simulink model "CEL_Lab1_Feedforward"  (R2024b)
settings: Solver=ode45  StartTime=0.0  StopTime=5
values from neighbouring files (symbols this model uses):
  PID = computePIDGains(8, 0.15, 0.1, plant.Ps, "PID")    [lab1_startup.m]
undefined symbols (not defined in the file or in its folder): drv, gbox, mld, mot, rads2rpm, sens
libraries: simulink_extras x3
settings Model: Creator=bmm1  LastModifiedBy=bmm1
settings RTWCC: GPUComputeCapability=3.5

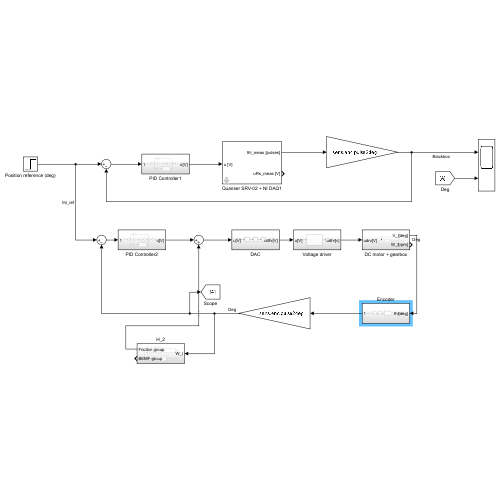
[thumbnail: Simulink's stored preview of the top-level diagram]
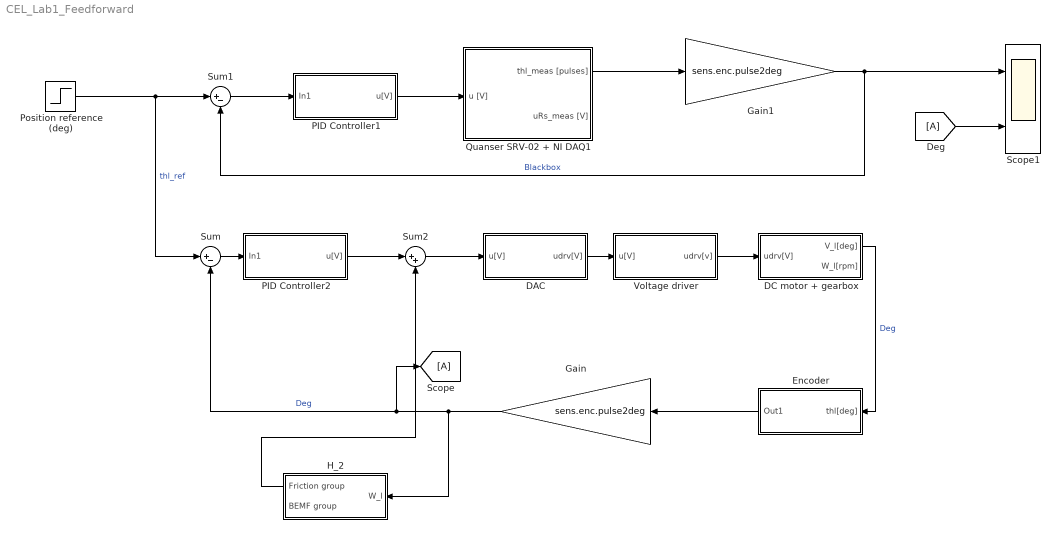
== system CEL_Lab1_Feedforward ==
  DAC : Subsystem
  DC motor + gearbox : Subsystem
  Deg : From
  Encoder : Subsystem
  Gain : Gain  Gain=sens.enc.pulse2deg
  Gain1 : Gain  Gain=sens.enc.pulse2deg
  H_2 : Subsystem
  PID Controller1 : Subsystem
  PID Controller2 : Subsystem
  Position reference (deg) : Step  Time=0.5  After=360  SampleTime=0
  Quanser SRV-02 + NI DAQ1 : Subsystem  mask(Quanser SRV-02 (with inertial load) + NI DAQ){Ts=0.001, fricType=Coulomb + viscous}
      mask prompts: Ts "NI DAQ Sample Time:"; fricType "Friction model"
      mask help: Quanser SRV-02 (with inertial load) + NI DAQ model.
      mask init:
      | %%  Sensors data
      | 
      | %   shunt resistor
      | sens.curr.Rs = 0.5;                         %   resistance [Ohm]   
      | sens.curr.uRs_std = 0.01;                   %   voltage noise standard dev [V]                           
      | sens.curr.uRs_var = sens.curr.uRs_std^2;	%   voltage noise variance [V^2]
      | 
      | %   Hewlett-Packard HEDS-5540#A06 optical encoder
      | sens.enc.ppr = 500*4;                       %   pulses per rotation
      | sens.enc.pulse2deg = 360/sens.enc.ppr;      %   [pulses] -> [deg]
      | sens.enc.pulse2rad = 2*pi/sens.enc.ppr;     %   [pulses] -> [rad]
      | sens.enc.deg2pulse = sens.enc.ppr/360;      %   [deg] -> [pulses]
      | sens.enc.rad2pulse = sens.enc.ppr/2/pi;     %   [rad] -> [pulses]
      | 
      | 
      | %%  Data acquisition board (daq) data
      | 
      | %   NI PCI-6221 DAC data
      | daq.dac.bits = 16;                                  %   resolution (bits)
      | daq.dac.fs   = 10;                                  %   full scale 
      | daq.dac.q    = 2*daq.dac.fs/(2^daq.dac.bits-1);     %	quantization
      | 
      | %   NI PCI-6221 ADC data
      | daq.adc.bits = 16;                                  %   resolution (bits)
      | daq.adc.fs   = 10;                                  %   full scale (as set in SLDRT Analog Input block)
      | daq.adc.q    = 2*daq.adc.fs/(2^daq.adc.bits-1);     %   quantization
      mask Help:
      | Riccardo Antonello (antonello@dei.unipd.it)
      | 
      | April 24, 2020
      | 
      | Dept. of Information Engineering, University of Padova
      mask TypeOptions fricType: Coulomb + viscous | Karnopp
  Scope : Goto
  Scope1 : Scope  NumInputPorts=2
  Sum : Sum  Inputs=|+-
  Sum1 : Sum  Inputs=|+-
  Sum2 : Sum  Inputs=|++
  Voltage driver : Subsystem
  wires:
  Position reference (deg)/1 -> Sum/1, Sum1/1  "thl_ref"
  Gain/1 -> H_2/1(W_l), Sum/2, Scope/1  "Deg"
  Sum/1 -> PID Controller2/1(In1)
  DAC/1(udrv[V]) -> Voltage driver/1(u[V])
  Voltage driver/1(udrv[v]) -> DC motor + gearbox/1(udrv[V])
  DC motor + gearbox/1(V_l[deg]) -> Encoder/1(thl[deg])  "Deg"
  Quanser SRV-02 + NI DAQ1/1(thl_meas [pulses]) -> Gain1/1
  Gain1/1 -> Sum1/2, Scope1/1  "Blackbox"
  PID Controller1/1(u[V]) -> Quanser SRV-02 + NI DAQ1/1(u [V])
  Sum1/1 -> PID Controller1/1(In1)
  Encoder/1(Out1) -> Gain/1
  Deg/1 -> Scope1/2
  PID Controller2/1(u[V]) -> Sum2/1
  Sum2/1 -> DAC/1(u[V])
  H_2/1(Friction group) -> Sum2/2

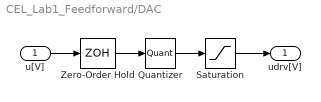
== system CEL_Lab1_Feedforward/DAC ==
  u[V] : Inport
  Quantizer : Quantizer  QuantizationInterval=daq.dac.q
  Saturation : Saturate  UpperLimit=10  LowerLimit=-10
  Zero-Order Hold : ZeroOrderHold  SampleTime=1e-3
  udrv[V] : Outport
  wires:
  Zero-Order Hold/1 -> Quantizer/1
  u[V]/1 -> Zero-Order Hold/1
  Quantizer/1 -> Saturation/1
  Saturation/1 -> udrv[V]/1

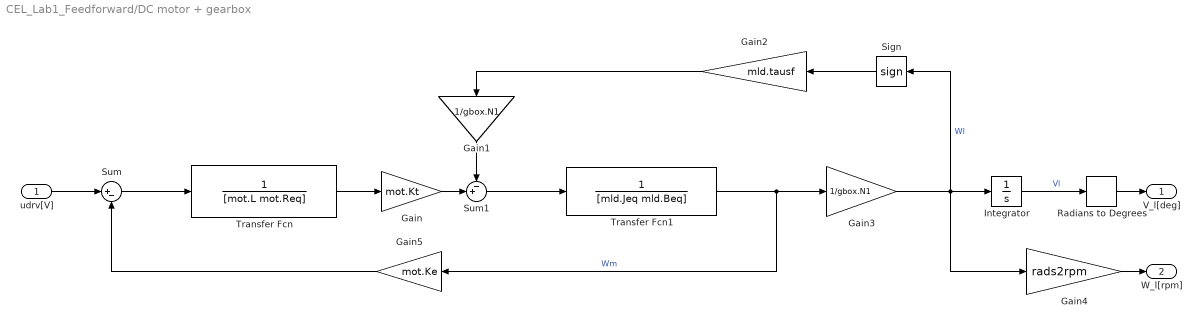
== system CEL_Lab1_Feedforward/DC motor + gearbox ==
  udrv[V] : Inport
  Gain : Gain  Gain=mot.Kt
  Gain1 : Gain  Gain=1/gbox.N1
  Gain2 : Gain  Gain=mld.tausf
  Gain3 : Gain  Gain=1/gbox.N1
  Gain4 : Gain  Gain=rads2rpm
  Gain5 : Gain  Gain=mot.Ke
  Integrator : Integrator
  Radians to Degrees : simulink_extras/Transformations/Radians to Degrees
  Sign : Signum  ZeroCross=off
  Sum : Sum  Inputs=|+-
  Sum1 : Sum  Inputs=-+|
  Transfer Fcn : TransferFcn  Denominator=[mot.L mot.Req]
  Transfer Fcn1 : TransferFcn  Denominator=[mld.Jeq mld.Beq]
  V_l[deg] : Outport
  W_l[rpm] : Outport  Port=2
  wires:
  udrv[V]/1 -> Sum/1
  Sum/1 -> Transfer Fcn/1
  Transfer Fcn/1 -> Gain/1
  Gain1/1 -> Sum1/1
  Gain2/1 -> Gain1/1
  Sign/1 -> Gain2/1
  Transfer Fcn1/1 -> Gain5/1, Gain3/1  "Wm"
  Gain3/1 -> Gain4/1, Sign/1, Integrator/1  "Wl"
  Integrator/1 -> Radians to Degrees/1  "Vl"
  Radians to Degrees/1 -> V_l[deg]/1
  Gain4/1 -> W_l[rpm]/1
  Sum1/1 -> Transfer Fcn1/1
  Gain/1 -> Sum1/2
  Gain5/1 -> Sum/2

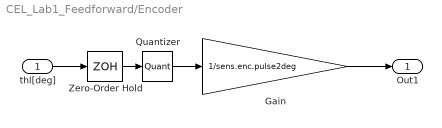
== system CEL_Lab1_Feedforward/Encoder ==
  thl[deg] : Inport
  Gain : Gain  Gain=1/sens.enc.pulse2deg
  Quantizer : Quantizer  QuantizationInterval=sens.enc.pulse2deg
  Zero-Order Hold : ZeroOrderHold  SampleTime=1e-3
  Out1 : Outport
  wires:
  thl[deg]/1 -> Zero-Order Hold/1
  Gain/1 -> Out1/1
  Quantizer/1 -> Gain/1
  Zero-Order Hold/1 -> Quantizer/1

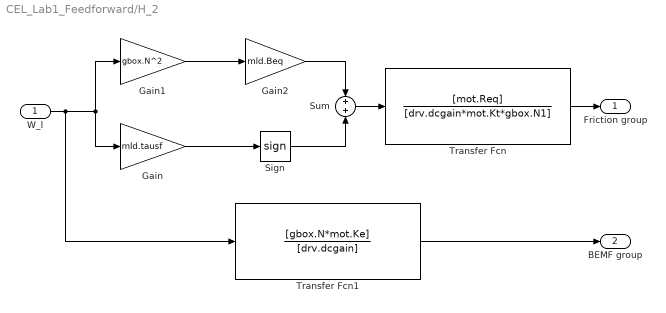
== system CEL_Lab1_Feedforward/H_2 ==
  W_l : Inport
  Gain : Gain  Gain=mld.tausf
  Gain1 : Gain  Gain=gbox.N^2
  Gain2 : Gain  Gain=mld.Beq
  Sign : Signum
  Sum : Sum  Inputs=+|+
  Transfer Fcn : TransferFcn  Numerator=[mot.Req]  Denominator=[drv.dcgain*mot.Kt*gbox.N1]
  Transfer Fcn1 : TransferFcn  Numerator=[gbox.N*mot.Ke]  Denominator=[drv.dcgain]
  Friction group : Outport
  BEMF group : Outport  Port=2
  wires:
  W_l/1 -> Transfer Fcn1/1, Gain1/1, Gain/1
  Gain/1 -> Sign/1
  Gain1/1 -> Gain2/1
  Sign/1 -> Sum/2
  Gain2/1 -> Sum/1
  Sum/1 -> Transfer Fcn/1
  Transfer Fcn/1 -> Friction group/1
  Transfer Fcn1/1 -> BEMF group/1

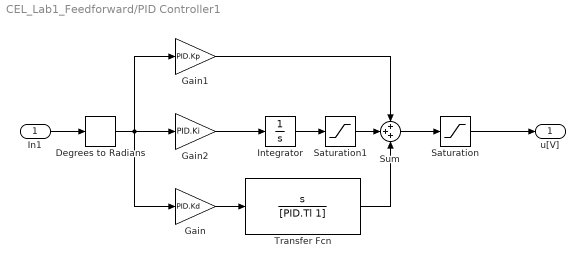
== system CEL_Lab1_Feedforward/PID Controller1 ==
  In1 : Inport
  Degrees to Radians : simulink_extras/Transformations/Degrees to Radians
  Gain : Gain  Gain=PID.Kd
  Gain1 : Gain  Gain=PID.Kp
  Gain2 : Gain  Gain=PID.Ki
  Integrator : Integrator
  Saturation : Saturate  UpperLimit=10  LowerLimit=-10
  Saturation1 : Saturate  UpperLimit=PID.i_saturation  LowerLimit=-PID.i_saturation
  Sum : Sum  Inputs=+++
  Transfer Fcn : TransferFcn  Numerator=[1 0]  Denominator=[PID.Tl 1]
  u[V] : Outport
  wires:
  In1/1 -> Degrees to Radians/1
  Sum/1 -> Saturation/1
  Saturation/1 -> u[V]/1
  Degrees to Radians/1 -> Gain/1, Gain1/1, Gain2/1
  Gain/1 -> Transfer Fcn/1
  Gain2/1 -> Integrator/1
  Transfer Fcn/1 -> Sum/3
  Integrator/1 -> Saturation1/1
  Gain1/1 -> Sum/1
  Saturation1/1 -> Sum/2

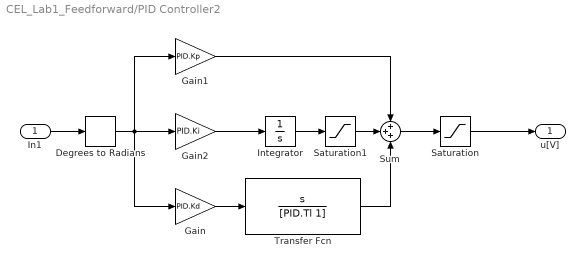
== system CEL_Lab1_Feedforward/PID Controller2 ==
  In1 : Inport
  Degrees to Radians : simulink_extras/Transformations/Degrees to Radians
  Gain : Gain  Gain=PID.Kd
  Gain1 : Gain  Gain=PID.Kp
  Gain2 : Gain  Gain=PID.Ki
  Integrator : Integrator
  Saturation : Saturate  UpperLimit=10  LowerLimit=-10
  Saturation1 : Saturate  UpperLimit=PID.i_saturation  LowerLimit=-PID.i_saturation
  Sum : Sum  Inputs=+++
  Transfer Fcn : TransferFcn  Numerator=[1 0]  Denominator=[PID.Tl 1]
  u[V] : Outport
  wires:
  In1/1 -> Degrees to Radians/1
  Sum/1 -> Saturation/1
  Saturation/1 -> u[V]/1
  Degrees to Radians/1 -> Gain/1, Gain1/1, Gain2/1
  Gain/1 -> Transfer Fcn/1
  Gain2/1 -> Integrator/1
  Transfer Fcn/1 -> Sum/3
  Integrator/1 -> Saturation1/1
  Gain1/1 -> Sum/1
  Saturation1/1 -> Sum/2

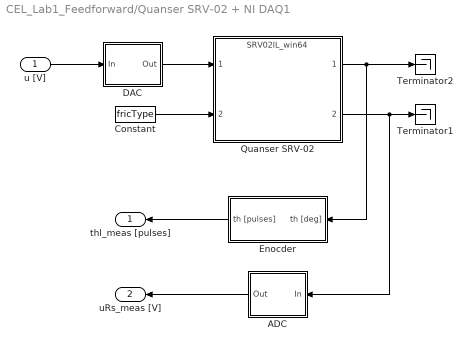
== system CEL_Lab1_Feedforward/Quanser SRV-02 + NI DAQ1 ==
  u [V] : Inport
  ADC : Subsystem
  Constant : Constant  Value=fricType
  DAC : Subsystem
  Enocder : Subsystem
  Quanser SRV-02 : ModelReference  ModelNameDialog=SRV02IL_win64.slxp  ModelReferenceVersion=1.44  CopyOfModelProtected=on
  Terminator1 : Terminator
  Terminator2 : Terminator
  thl_meas [pulses] : Outport
  uRs_meas [V] : Outport  Port=2
  wires:
  Enocder/1(th [pulses]) -> thl_meas [pulses]/1
  ADC/1(Out) -> uRs_meas [V]/1
  DAC/1(Out) -> Quanser SRV-02/1
  Quanser SRV-02/2 -> ADC/1(In), Terminator1/1
  u [V]/1 -> DAC/1(In)
  Quanser SRV-02/1 -> Enocder/1(th [deg]), Terminator2/1
  Constant/1 -> Quanser SRV-02/2

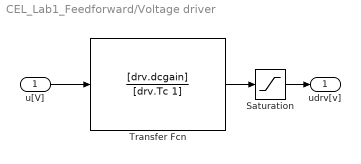
== system CEL_Lab1_Feedforward/Voltage driver ==
  u[V] : Inport
  Saturation : Saturate  UpperLimit=12  LowerLimit=-12
  Transfer Fcn : TransferFcn  Numerator=[drv.dcgain]  Denominator=[drv.Tc 1]
  udrv[v] : Outport
  wires:
  u[V]/1 -> Transfer Fcn/1
  Transfer Fcn/1 -> Saturation/1
  Saturation/1 -> udrv[v]/1

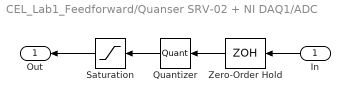
== system CEL_Lab1_Feedforward/Quanser SRV-02 + NI DAQ1/ADC ==
  In : Inport
  Quantizer : Quantizer  QuantizationInterval=daq.adc.q
  Saturation : Saturate  UpperLimit=daq.adc.fs  LowerLimit=-daq.adc.fs
  Zero-Order Hold : ZeroOrderHold  SampleTime=Ts
  Out : Outport
  wires:
  Saturation/1 -> Out/1
  In/1 -> Zero-Order Hold/1
  Quantizer/1 -> Saturation/1
  Zero-Order Hold/1 -> Quantizer/1

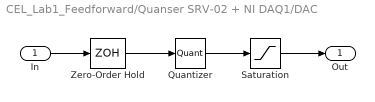
== system CEL_Lab1_Feedforward/Quanser SRV-02 + NI DAQ1/DAC ==
  In : Inport
  Quantizer : Quantizer  QuantizationInterval=daq.dac.q
  Saturation : Saturate  UpperLimit=daq.dac.fs  LowerLimit=-daq.dac.fs
  Zero-Order Hold : ZeroOrderHold  SampleTime=Ts
  Out : Outport
  wires:
  Quantizer/1 -> Saturation/1
  In/1 -> Zero-Order Hold/1
  Zero-Order Hold/1 -> Quantizer/1
  Saturation/1 -> Out/1

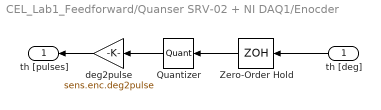
== system CEL_Lab1_Feedforward/Quanser SRV-02 + NI DAQ1/Enocder ==
  th [deg] : Inport
  Quantizer : Quantizer  QuantizationInterval=sens.enc.pulse2deg
  Zero-Order Hold : ZeroOrderHold  SampleTime=Ts
  deg2pulse : Gain  Gain=sens.enc.deg2pulse
  th [pulses] : Outport
  wires:
  Quantizer/1 -> deg2pulse/1
  th [deg]/1 -> Zero-Order Hold/1
  Zero-Order Hold/1 -> Quantizer/1
  deg2pulse/1 -> th [pulses]/1
